simulink model "delay_bram_prog_dp_blk"  (R2019a)
settings: Solver=VariableStepAuto  StartTime=0.0  StopTime=20.0  RelTol=1e-3
libraries: xbsIndex_r4 x1
settings Model: Creator=mybur  LastModifiedBy=mybur

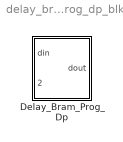
== system delay_bram_prog_dp_blk ==
  Delay_Bram_Prog_Dp : Subsystem  mask{max_delay=4, bram_latency=2, bram_primitive="block", is_async=off}
      mask prompts: max_delay "Max Delay (2^?)"; bram_latency "BRAM Latency"; bram_primitive "BRAM Primitive"; is_async "Is Asynchronous?"
      mask init:
      | Simulink.Block.eval([gcb, '/delay_bram_prog_dp']);
      | 
      | knit_subsystem_to_blackbox('delay_bram_prog_dp');
      mask TypeOptions bram_primitive: "block" | "distributed" | "auto" | "ultra"
      mask DialogControl DescTextVar Prompt: A delay module that uses a dual port BRAM to delay the input by the delay period provided.

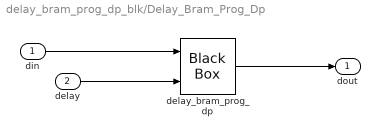
== system delay_bram_prog_dp_blk/Delay_Bram_Prog_Dp ==
  din : Inport
  delay : Inport  Port=2
  delay_bram_prog_dp : xbsIndex_r4/Black Box  init_code=delay_bram_prog_dp_config  sim_method=ISE Simulator  verbose=off  block_type=blackbox2
  dout : Outport
  wires:
  din/1 -> delay_bram_prog_dp/1
  delay/1 -> delay_bram_prog_dp/2
  delay_bram_prog_dp/1 -> dout/1
